simulink model "UVelocityIOLoopSystem"  (R2020a)
settings: Solver=VariableStepAuto  StartTime=0.0  StopTime=10.0  RelTol=1e-3
settings Model: Creator=OZAN  LastModifiedBy=OZAN

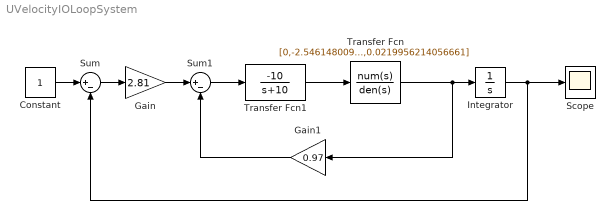
== system UVelocityIOLoopSystem ==
  Constant : Constant
  Gain : Gain  Gain=2.81
  Gain1 : Gain  Gain=0.97
  Integrator : Integrator
  Scope : Scope
  Sum : Sum  Inputs=|+-
  Sum1 : Sum  Inputs=|+-
  Transfer Fcn : TransferFcn  Numerator=[0,-2.54614800990840,0]  Denominator=[1,0.0683145596084275,0.0219956214056661]
  Transfer Fcn1 : TransferFcn  Numerator=[-10]  Denominator=[1 10]
  wires:
  Sum/1 -> Gain/1
  Integrator/1 -> Scope/1, Sum/2
  Gain/1 -> Sum1/1
  Sum1/1 -> Transfer Fcn1/1
  Transfer Fcn/1 -> Gain1/1, Integrator/1
  Transfer Fcn1/1 -> Transfer Fcn/1
  Gain1/1 -> Sum1/2
  Constant/1 -> Sum/1
